simulink library "usask_tlm_lib"  (R2015a)
settings: Solver=ode45  SolverMode=SingleTasking  StartTime=0.0  StopTime=10.0  RelTol=1e-3
undefined symbols (not defined in the file): B, d, L, m_E, m_G, nu, rho
libraries: TaperedTLMElasticLib x8, transmission_lines x2
(part 1 of 2)
settings Model: Creator=tkw954  LastModifiedBy=Jeremy
settings DataIOCC: SignalLoggingSaveFormat=ModelDataLogs
settings OptimizationCC: BlockReduction=off  BooleanDataType=off
settings DebuggingCC: SaveWithParameterizedLinksMsg=none  UnderspecifiedInitializationDetection=Classic  MergeDetectMultiDrivingBlocksExec=none  SignalResolutionControl=TryResolveAllWithWarning  MultiTaskDSMMsg=warning  MultiTaskCondExecSysMsg=none  StateNameClashWarn=warning  StrictBusMsg=None
settings HardwareCC: TargetUnknown=on

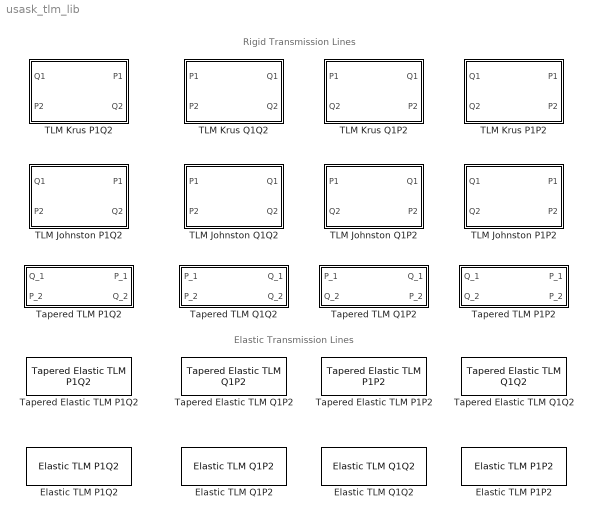
== system usask_tlm_lib ==
  note: Elastic Transmission Lines
  note: Rigid Transmission Lines
  Elastic TLM P1P2 : TaperedTLMElasticLib/Elastic TLM P1P2  K=1.5e9  nu=100e-6  rho=890  D=42e-3  L=10  e_pipe=6e-3  E=190e9  nu_p=0.3  axial_effect=Anchored throughout
  Elastic TLM P1Q2 : TaperedTLMElasticLib/Elastic TLM P1Q2  K=1.5e9  nu=100e-6  rho=890  D=42e-3  L=10  e_pipe=6e-3  E=190e9  nu_p=0.3  axial_effect=Anchored throughout
  Elastic TLM Q1P2 : TaperedTLMElasticLib/Elastic TLM Q1P2  K=1.5e9  nu=100e-6  rho=890  D=42e-3  L=10  e_pipe=6e-3  E=190e9  nu_p=0.3  axial_effect=Anchored throughout
  Elastic TLM Q1Q2 : TaperedTLMElasticLib/Elastic TLM Q1Q2  K=1.5e9  nu=100e-6  rho=890  D=42e-3  L=10  e_pipe=6e-3  E=190e9  nu_p=0.3  axial_effect=Anchored throughout
  TLM Johnston P1P2 : Subsystem  mask(Transmission Line){L=L, d=d, rho=rho, nu=nu, B=B, modelNumber=2, useCorrected=on}
      mask prompts: L "Length (m)"; d "Diameter (m)"; rho "Density (kg/m^3)"; nu "Kinematic viscosity (m^2/s)"; B "Bulk Modulus (Pa)"; modelNumber "Model Number"; useCorrected "Use corrected impedence"
      mask help:
      | Calculates pipeline dynamics using the Transmission Line Method (TLM).
      |
      | This implementation follows Johnston (2012), which includes an approximation of unsteady laminar flow and frequency-dependent velocity profile. It neglects thermal effects and assumes zero initial pressure and flow.
      |
      | Three models are implemented. Model 1 may be unstable for high beta (see paper). Model 2 is recommended.
      |
      | One may choose to use a more complicated impedence model to compensate for errors in capacitance.
      |
      | Positive flows are into both ports.
      |
      | Reference
      | Johnston, Nigel. "The transmission line method for modelling laminar flow of liquid in pipelines." Proceedings of the Institution of Mechanical Engineers, Part I: Journal of Systems and Control Engineering 226.5 (2012): 586-597.
      mask init:
      | c=sqrt(B/rho);%(m/s) sonic speed
      | 
      | A=pi/4*d^2;%(m^2) cross sectional area
      | r=d/2;%(m) radius
      | T=L/c;%(s) propagation time
      | 
      | R=8*rho*nu*L/(pi*r^4);%(Pa/(m^3/s)) Resistance
      | 
      | K=1.25;%empirical constant
      | 
      | beta=nu*T/r^2;%dissipation number
      | fprintf('beta=%f\n',beta);
      | 
      | k=4;%this must match order of G2 diagram
      | m=nan(k,1);
      | m(1)=2.2457;
      | if k>1
      | m(2)=6.8400;
      | end
      | for i=3:k
      |     m(i)=3*m(i-1);
      | end
      | 
      | 
      | n=nan(k,1);
      | n(1)=42.849;
      | for i=2:k
      |     n(i)=9*n(i-1);
      | end
      | 
      | if useCorrected
      |     Zc=rho*c/A*(1+K*(1-exp(-4*beta))+2*sum(m./n)-4*beta);%(Pa/(m^3/s)) impedence
      | else
      |     Zc=rho*c/A;%(Pa/(m^3/s)) impedence
      | end
      mask TypeOptions modelNumber: 1 | 2 | 3
  TLM Johnston P1Q2 : Subsystem  mask(Transmission Line){L=45, d=13e-3, rho=870, nu=1.2402e-04, B=1.5182e9, modelNumber=2, useCorrected=on}
      mask prompts: L "Length (m)"; d "Diameter (m)"; rho "Density (kg/m^3)"; nu "Kinematic viscosity (m^2/s)"; B "Bulk Modulus (Pa)"; modelNumber "Model Number"; useCorrected "Use corrected impedence"
      mask help:
      | Calculates pipeline dynamics using the Transmission Line Method (TLM).
      |
      | This implementation follows Johnston (2012), which includes an approximation of unsteady laminar flow and frequency-dependent velocity profile. It neglects thermal effects and assumes zero initial pressure and flow.
      |
      | Three models are implemented. Model 1 may be unstable for high beta (see paper). Model 2 is recommended.
      |
      | One may choose to use a more complicated impedence model to compensate for errors in capacitance.
      |
      | Positive flows are into both ports.
      |
      | Reference
      | Johnston, Nigel. "The transmission line method for modelling laminar flow of liquid in pipelines." Proceedings of the Institution of Mechanical Engineers, Part I: Journal of Systems and Control Engineering 226.5 (2012): 586-597.
      mask init: same as usask_tlm_lib/TLM Johnston P1P2
      mask TypeOptions modelNumber: 1 | 2 | 3
  TLM Johnston Q1P2 : Subsystem  mask(Transmission Line){L=45, d=13e-3, rho=870, nu=1.2402e-04, B=1.5182e9, modelNumber=2, useCorrected=on}
      mask prompts: L "Length (m)"; d "Diameter (m)"; rho "Density (kg/m^3)"; nu "Kinematic viscosity (m^2/s)"; B "Bulk Modulus (Pa)"; modelNumber "Model Number"; useCorrected "Use corrected impedence"
      mask help:
      | Calculates pipeline dynamics using the Transmission Line Method (TLM).
      |
      | This implementation follows Johnston (2012), which includes an approximation of unsteady laminar flow and frequency-dependent velocity profile. It neglects thermal effects and assumes zero initial pressure and flow.
      |
      | Three models are implemented. Model 1 may be unstable for high beta (see paper). Model 2 is recommended.
      |
      | One may choose to use a more complicated impedence model to compensate for errors in capacitance.
      |
      | Positive flows are into both ports.
      |
      | Reference
      | Johnston, Nigel. "The transmission line method for modelling laminar flow of liquid in pipelines." Proceedings of the Institution of Mechanical Engineers, Part I: Journal of Systems and Control Engineering 226.5 (2012): 586-597.
      mask init: same as usask_tlm_lib/TLM Johnston P1P2
      mask TypeOptions modelNumber: 1 | 2 | 3
  TLM Johnston Q1Q2 : Subsystem  mask(Transmission Line){L=45, d=13e-3, rho=870, nu=1.2402e-04, B=1.5182e9, modelNumber=2, useCorrected=on}
      mask prompts: L "Length (m)"; d "Diameter (m)"; rho "Density (kg/m^3)"; nu "Kinematic viscosity (m^2/s)"; B "Bulk Modulus (Pa)"; modelNumber "Model Number"; useCorrected "Use corrected impedence"
      mask help:
      | Calculates pipeline dynamics using the Transmission Line Method (TLM).
      |
      | This implementation follows Johnston (2012), which includes an approximation of unsteady laminar flow and frequency-dependent velocity profile. It neglects thermal effects and assumes zero initial pressure and flow.
      |
      | Three models are implemented. Model 1 may be unstable for high beta (see paper). Model 2 is recommended.
      |
      | One may choose to use a more complicated impedence model to compensate for errors in capacitance.
      |
      | Positive flows are into both ports.
      |
      | Reference
      | Johnston, Nigel. "The transmission line method for modelling laminar flow of liquid in pipelines." Proceedings of the Institution of Mechanical Engineers, Part I: Journal of Systems and Control Engineering 226.5 (2012): 586-597.
      mask init: same as usask_tlm_lib/TLM Johnston P1P2
      mask TypeOptions modelNumber: 1 | 2 | 3
  TLM Krus P1P2 : Subsystem  mask(Transmission Line){L=45, d=13e-3, rho=870, nu=1.2402e-04, B=1.5182e9}
      mask prompts: L "Length (m)"; d "Diameter (m)"; rho "Density (kg/m^3)"; nu "Kinematic viscosity (m^2/s)"; B "Bulk Modulus (Pa)"
      mask help:
      | Calculates pipeline dynamics using the Transmission Line Method (TLM).
      |
      | This implementation follows Krus et al (1994), which neglects unsteady friciton and uses simple transfer functions for the filters.
      |
      | Reference
      | Krus P, Weddfelt K and Palmberg J-O. Fast pipeline models for simulation of hydraulic systems. J Dyn Syst Measure Control 1994; 116(1): 132–136.
      mask init:
      | c=sqrt(B/rho);%(m/s) sonic speed
      | 
      | A=pi/4*d^2;%(m^2) cross sectional area
      | r=d/2;%(m) radius
      | T=L/c;%(s) propagation time
      | 
      | R=8*rho*nu*L/(pi*r^4);%(Pa/(m^3/s)) Resistance
      | 
      | K=1.25;%empirical constant
      | 
      | Zc=rho*c/A;%(Pa/(m^3/s)) impedence
      | 
      | beta=nu*T/r^2;%dissipation number
      | fprintf('beta=%f\n',beta);
  TLM Krus P1Q2 : Subsystem  mask(Transmission Line){L=45, d=13e-3, rho=870, nu=1.2402e-04, B=1.5182e9}
      mask prompts: L "Length (m)"; d "Diameter (m)"; rho "Density (kg/m^3)"; nu "Kinematic viscosity (m^2/s)"; B "Bulk Modulus (Pa)"
      mask help:
      | Calculates pipeline dynamics using the Transmission Line Method (TLM).
      |
      | This implementation follows Krus et al (1994), which neglects unsteady friciton and uses simple transfer functions for the filters.
      |
      | Reference
      | Krus P, Weddfelt K and Palmberg J-O. Fast pipeline models for simulation of hydraulic systems. J Dyn Syst Measure Control 1994; 116(1): 132–136.
      mask init: same as usask_tlm_lib/TLM Krus P1P2
  TLM Krus Q1P2 : Subsystem  mask(Transmission Line){L=45, d=13e-3, rho=870, nu=1.2402e-04, B=1.5182e9}
      mask prompts: L "Length (m)"; d "Diameter (m)"; rho "Density (kg/m^3)"; nu "Kinematic viscosity (m^2/s)"; B "Bulk Modulus (Pa)"
      mask help:
      | Calculates pipeline dynamics using the Transmission Line Method (TLM).
      |
      | This implementation follows Krus et al (1994), which neglects unsteady friciton and uses simple transfer functions for the filters.
      |
      | Reference
      | Krus P, Weddfelt K and Palmberg J-O. Fast pipeline models for simulation of hydraulic systems. J Dyn Syst Measure Control 1994; 116(1): 132–136.
      mask init: same as usask_tlm_lib/TLM Krus P1P2
  TLM Krus Q1Q2 : Subsystem  mask(Transmission Line){L=45, d=13e-3, rho=870, nu=1.2402e-04, B=1.5182e9}
      mask prompts: L "Length (m)"; d "Diameter (m)"; rho "Density (kg/m^3)"; nu "Kinematic viscosity (m^2/s)"; B "Bulk Modulus (Pa)"
      mask help:
      | Calculates pipeline dynamics using the Transmission Line Method (TLM).
      |
      | This implementation follows Krus et al (1994), which neglects unsteady friciton and uses simple transfer functions for the filters.
      |
      | Reference
      | Krus P, Weddfelt K and Palmberg J-O. Fast pipeline models for simulation of hydraulic systems. J Dyn Syst Measure Control 1994; 116(1): 132–136.
      mask init: same as usask_tlm_lib/TLM Krus P1P2
  Tapered Elastic TLM P1P2 : TaperedTLMElasticLib/Tapered Elastic TLM P1P2  K=1.5e9  nu=100e-6  rho=890  D_1=40e-3  D_2=42e-3  L=10  e_pipe=3e-3  E=2e9  nu_p=0.3  axial_effect=Anchored throughout
  Tapered Elastic TLM P1Q2 : TaperedTLMElasticLib/Tapered Elastic TLM P1Q2  K=1.5e9  nu=100e-6  rho=890  D_1=40e-3  D_2=42e-3  L=10  e_pipe=3e-3  E=2e9  nu_p=0.3  axial_effect=Anchored throughout
  Tapered Elastic TLM Q1P2 : TaperedTLMElasticLib/Tapered Elastic TLM Q1P2  K=1.5e9  nu=100e-6  rho=890  D_1=40e-3  D_2=42e-3  L=10  e_pipe=3e-3  E=2e9  nu_p=0.3  axial_effect=Anchored throughout
  Tapered Elastic TLM Q1Q2 : TaperedTLMElasticLib/Tapered Elastic TLM Q1Q2  K=1.5e9  nu=100e-6  rho=890  D_1=40e-3  D_2=42e-3  L=10  e_pipe=3e-3  E=2e9  nu_p=0.3  axial_effect=Anchored throughout
  Tapered TLM P1P2 : Subsystem  mask(Tapered Hydraulic Transmission Line (TLM)){D_1=40e-3, D_2=42e-3, L=10, K=1.5e9, nu=100e-6, rho=890}
      mask prompts: D_1 "Inlet Diameter (m)"; D_2 "Outlet Diameter (m)"; L "Length (m)"; K "Oil Bulk Modulus (Pa)"; nu "Oil Viscosity (m^2/s)"; rho "Oil Density (kg/m^3)"
      mask help:
      | This model implements the transmission line model in ven der Buhs and Wiens (2017). The method uses the the transfer function form from Johnston et. al (2014), however the weighting factors are determined from an optimization procedure comparing to the exact transmission matrix for a tapered pipeline.
      |
      | This model assumes a rigid-walled tube with a linear taper in radius between the two ports. It assumes constant bulk modulus (no cavitation or entrined air effects) and includes frequency-dependent friction effects.
      |
      | Positive flows are directed into either port.
      |
      | This model also assumes zero initial conditions
      |
      | Reference:
      | N Johnston, M Pan, and S Kudzma. An enhanced transmission line method for modelling laminar flow of liquid in pipelines. Journal of Systems and Control Engineering, 228(4):193–206, 2014.
      |
      | J ven der Buhs and T Wiens. Modelling Dynamic Response of Hydraulic Fluid Within Tapered Transmission Lines. Proceedings of the 15th Scandinavian International Conference on Fluid Power, 2017
      mask init:
      | %% Note: Equation numbers from:
      | % J ven der Buhs and T Wiens. Modelling Dynamic Response of Hydraulic Fluid Within Tapered 
      | % Transmission Lines. Proceedings of the 15th Scandinavian International Conference on Fluid 
      | % Power, Linköping University, Sweden, 2017.
      | %%
      | 
      | % Check for positive params, report error if negative given
      | if D_1<0 | D_2<0 | L<0 | K<0 | nu<0 | rho<0
      |     error('Please ensure parameters are all positive')
      | end
      | 
      | r1 = D_1/2; % Inlet radius (m)
      | r2 = D_2/2; % Outlet radius (m)
      | 
      | c=sqrt(K/rho);% Local speed of sound (m/s)
      | lambda = min(r1,r2)/max(r1,r2); % Taper ratio (dimensionless), Equation (11)
      | beta = ((nu*L)/(c*max(r1,r2)^2))*((lambda^2+lambda+1)^2/(9*lambda^3)); % Dissipation number (dimensionless), Equation (13)
      | Z_c = ((3*c*rho)/(pi*max(r1,r2)^2))/(lambda^2+lambda+1); % Characteristic impedance (Pa•s/m^3), Equation (10)
      | T=L/c; % Wave propagation time (s)
      | 
      | k=6; % Number of weighting factors
      | 
      | % Grab optimized weighting factors and parameters. Please see paper for
      | % more detail on how these parameters were found.
      | [ m_E, m_G, tau ] = interpolateTLMparams( beta, lambda, k);
      | 
      | if isnan(m_E(1)) | isnan(m_G(1)) | isnan(tau)
      |     error('The parameters you have entered are outside the working range of this model. Weighting factors cannot be found')
      | end  
      |     
      | T_prime = tau*T; % Modified wave propagation time (s), Equation (18) 
      | 
      | n=nan(1,k); % Weighting factor initialization
      | n(1)=0.3/(1+3*beta); % Equation (19)
      | for i=2:k
      |     n(i)=n(i-1)*3; % Equation (19)
      | end
      | 
      | b=1-8*beta/sum(m_E./n); % Equation (16)
      | 
      | %Error Checking
      | load TaperedTLMAcceptableErrorContour.mat
      | IN = inpolygon(lambda,beta,lambda_poly,beta_poly);
      | if ~IN
      |     warning('Dissipaton number (beta) and taper ratio (lambda) combination are outside the recommended range')
      | end
      | 
      | 
      | 
      | 
      | %% End of initialization
      mask Display:
      | port_label('input', 1 , '\itq_1', 'texmode', 'on')
      | port_label('input', 2 , '\itq_2', 'texmode', 'on')
      | port_label('output', 1 , '\itp_1', 'texmode', 'on')
      | port_label('output', 2 , '\itp_2', 'texmode', 'on')
  Tapered TLM P1Q2 : Subsystem  mask(Tapered Hydraulic Transmission Line (TLM)){D_1=40e-3, D_2=42e-3, L=10, K=1.5e9, nu=100e-6, rho=890}
      mask prompts: D_1 "Inlet Diameter (m)"; D_2 "Outlet Diameter (m)"; L "Length (m)"; K "Oil Bulk Modulus (Pa)"; nu "Oil Viscosity (m^2/s)"; rho "Oil Density (kg/m^3)"
      mask help:
      | This model implements the transmission line model in ven der Buhs and Wiens (2017). The method uses the the transfer function form from Johnston et. al (2014), however the weighting factors are determined from an optimization procedure comparing to the exact transmission matrix for a tapered pipeline.
      |
      | This model assumes a rigid-walled tube with a linear taper in radius between the two ports. It assumes constant bulk modulus (no cavitation or entrined air effects) and includes frequency-dependent friction effects.
      |
      | Positive flows are directed into either port. This model also assumes zero initial conditions.
      |
      | "p" is fluid pressure in pascals (Pa).
      | "q" is fluid flow in cubic meters per second (m^3/s).
      | "_1" indicates the inlet, and "_2" indicates the outlet.
      |
      | Reference:
      | N Johnston, M Pan, and S Kudzma. An enhanced transmission line method for modelling laminar flow of liquid in pipelines. Journal of Systems and Control Engineering, 228(4):193–206, 2014.
      |
      | J ven der Buhs and T Wiens. Modelling Dynamic Response of Hydraulic Fluid Within Tapered Transmission Lines. Proceedings of the 15th Scandinavian International Conference on Fluid Power, Linköping University, Sweden, 2017.
      mask init: same as usask_tlm_lib/Tapered TLM P1P2
      mask Display:
      | port_label('input', 1 , '\itq_1', 'texmode', 'on')
      | port_label('input', 2 , '\itp_2', 'texmode', 'on')
      | port_label('output', 1 , '\itp_1', 'texmode', 'on')
      | port_label('output', 2 , '\itq_2', 'texmode', 'on')
  Tapered TLM Q1P2 : Subsystem  mask(Tapered Hydraulic Transmission Line (TLM)){D_1=40e-3, D_2=42e-3, L=10, K=1.5e9, nu=100e-6, rho=890}
      mask prompts: D_1 "Inlet Diameter (m)"; D_2 "Outlet Diameter (m)"; L "Length (m)"; K "Oil Bulk Modulus (Pa)"; nu "Oil Viscosity (m^2/s)"; rho "Oil Density (kg/m^3)"
      mask help:
      | This model implements the transmission line model in ven der Buhs and Wiens (2017). The method uses the the transfer function form from Johnston et. al (2014), however the weighting factors are determined from an optimization procedure comparing to the exact transmission matrix for a tapered pipeline.
      |
      | This model assumes a rigid-walled tube with a linear taper in radius between the two ports. It assumes constant bulk modulus (no cavitation or entrined air effects) and includes frequency-dependent friction effects.
      |
      | Positive flows are directed into either port.
      |
      | This model also assumes zero initial conditions
      |
      | Reference:
      | N Johnston, M Pan, and S Kudzma. An enhanced transmission line method for modelling laminar flow of liquid in pipelines. Journal of Systems and Control Engineering, 228(4):193–206, 2014.
      |
      | J ven der Buhs and T Wiens. Modelling Dynamic Response of Hydraulic Fluid Within Tapered Transmission Lines. Proceedings of the 15th Scandinavian International Conference on Fluid Power, 2017
      mask init: same as usask_tlm_lib/Tapered TLM P1P2
      mask Display:
      | port_label('input', 1 , '\itp_1', 'texmode', 'on')
      | port_label('input', 2 , '\itq_2', 'texmode', 'on')
      | port_label('output', 1 , '\itq_1', 'texmode', 'on')
      | port_label('output', 2 , '\itp_2', 'texmode', 'on')
  Tapered TLM Q1Q2 : Subsystem  mask(Tapered Hydraulic Transmission Line (TLM)){D_1=40e-3, D_2=42e-3, L=10, K=1.5e9, nu=100e-6, rho=890}
      mask prompts: D_1 "Inlet Diameter (m)"; D_2 "Outlet Diameter (m)"; L "Length (m)"; K "Oil Bulk Modulus (Pa)"; nu "Oil Viscosity (m^2/s)"; rho "Oil Density (kg/m^3)"
      mask help:
      | This model implements the transmission line model in ven der Buhs and Wiens (2017). The method uses the the transfer function form from Johnston et. al (2014), however the weighting factors are determined from an optimization procedure comparing to the exact transmission matrix for a tapered pipeline.
      |
      | This model assumes a rigid-walled tube with a linear taper in radius between the two ports. It assumes constant bulk modulus (no cavitation or entrined air effects) and includes frequency-dependent friction effects.
      |
      | Positive flows are directed into either port.
      |
      | This model also assumes zero initial conditions
      |
      | Reference:
      | N Johnston, M Pan, and S Kudzma. An enhanced transmission line method for modelling laminar flow of liquid in pipelines. Journal of Systems and Control Engineering, 228(4):193–206, 2014.
      |
      | J ven der Buhs and T Wiens. Modelling Dynamic Response of Hydraulic Fluid Within Tapered Transmission Lines. Proceedings of the 15th Scandinavian International Conference on Fluid Power, 2017
      mask init: same as usask_tlm_lib/Tapered TLM P1P2
      mask Display:
      | port_label('input', 1 , '\itp_1', 'texmode', 'on')
      | port_label('input', 2 , '\itp_2', 'texmode', 'on')
      | port_label('output', 1 , '\itq_1', 'texmode', 'on')
      | port_label('output', 2 , '\itq_2', 'texmode', 'on')

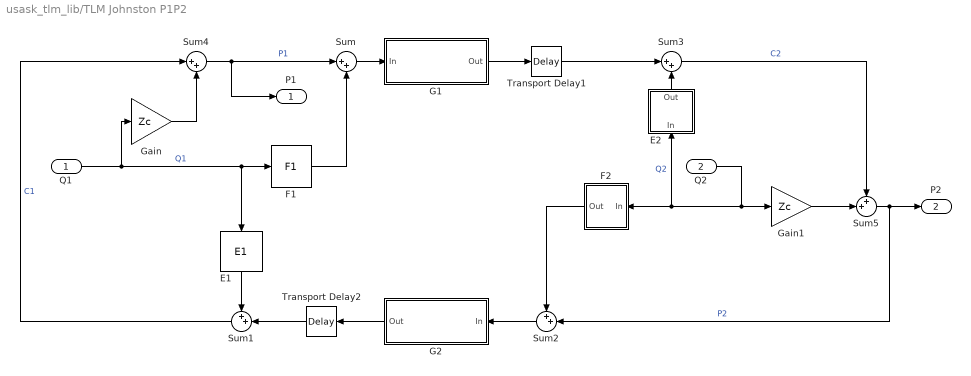
== system usask_tlm_lib/TLM Johnston P1P2 ==
  Q1 : Inport
  Q2 : Inport  Port=2
  E1 : transmission_lines/TLM Krus P1P2/E1
  E2 : Subsystem
  F1 : transmission_lines/TLM Krus P1P2/F1
  F2 : Subsystem
  G1 : Subsystem
  G2 : Subsystem
  Gain : Gain  Gain=Zc
  Gain1 : Gain  Gain=Zc
  Sum : Sum  Inputs=|++
  Sum1 : Sum  Inputs=++|
  Sum2 : Sum  Inputs=++|
  Sum3 : Sum  Inputs=|++
  Sum4 : Sum  Inputs=|++
  Sum5 : Sum  Inputs=++|
  Transport Delay1 : TransportDelay  DelayTime=T
  Transport Delay2 : TransportDelay  DelayTime=T
  P1 : Outport
  P2 : Outport  Port=2
  wires:
  Sum3/1 -> Sum5/1  "C2"
  G1/1(Out) -> Transport Delay1/1
  E2/1(Out) -> Sum3/2
  Sum5/1 -> Sum2/2, P2/1  "P2"
  Sum2/1 -> G2/1(In)
  F2/1(Out) -> Sum2/1
  Q2/1 -> F2/1(In), E2/1(In), Gain1/1  "Q2"
  Transport Delay1/1 -> Sum3/1
  Gain1/1 -> Sum5/2
  Sum/1 -> G1/1(In)
  Transport Delay2/1 -> Sum1/2
  Sum1/1 -> Sum4/1  "C1"
  F1/1 -> Sum/2
  E1/1 -> Sum1/1
  G2/1(Out) -> Transport Delay2/1
  Q1/1 -> Gain/1, F1/1, E1/1  "Q1"
  Sum4/1 -> P1/1, Sum/1  "P1"
  Gain/1 -> Sum4/2

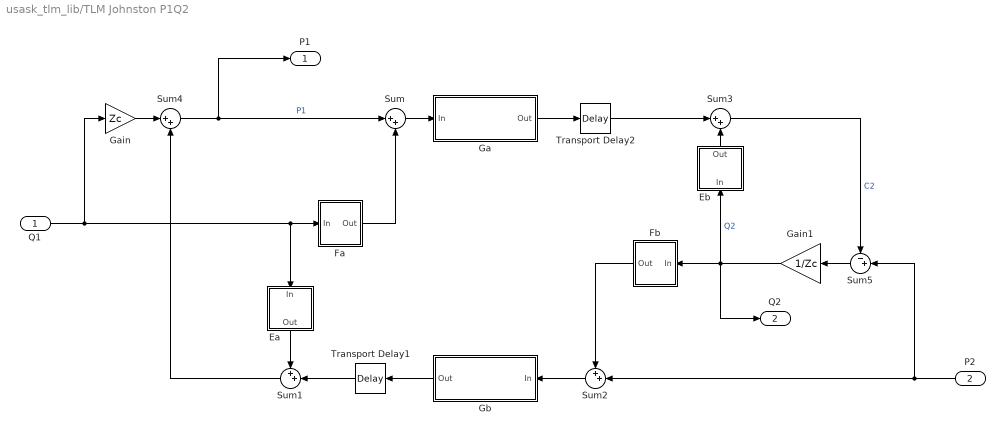
== system usask_tlm_lib/TLM Johnston P1Q2 ==
  Q1 : Inport
  P2 : Inport  Port=2
  Ea : Subsystem
  Eb : Subsystem
  Fa : Subsystem
  Fb : Subsystem
  Ga : Subsystem
  Gain : Gain  Gain=Zc
  Gain1 : Gain  Gain=1/Zc
  Gb : Subsystem
  Sum : Sum  Inputs=|++
  Sum1 : Sum  Inputs=++|
  Sum2 : Sum  Inputs=++|
  Sum3 : Sum  Inputs=|++
  Sum4 : Sum  Inputs=|++
  Sum5 : Sum  Inputs=-+|
  Transport Delay1 : TransportDelay  DelayTime=T
  Transport Delay2 : TransportDelay  DelayTime=T
  P1 : Outport
  Q2 : Outport  Port=2
  wires:
  Sum4/1 -> P1/1, Sum/1  "P1"
  Sum/1 -> Ga/1(In)
  Transport Delay2/1 -> Sum3/1
  Gain/1 -> Sum4/1
  Sum5/1 -> Gain1/1
  Transport Delay1/1 -> Sum1/2
  Q1/1 -> Gain/1, Ea/1(In), Fa/1(In)
  Sum1/1 -> Sum4/2
  Fa/1(Out) -> Sum/2
  Gain1/1 -> Q2/1, Eb/1(In), Fb/1(In)  "Q2"
  Fb/1(Out) -> Sum2/1
  Sum2/1 -> Gb/1(In)
  Ea/1(Out) -> Sum1/1
  Gb/1(Out) -> Transport Delay1/1
  P2/1 -> Sum5/2, Sum2/2
  Eb/1(Out) -> Sum3/2
  Ga/1(Out) -> Transport Delay2/1
  Sum3/1 -> Sum5/1  "C2"

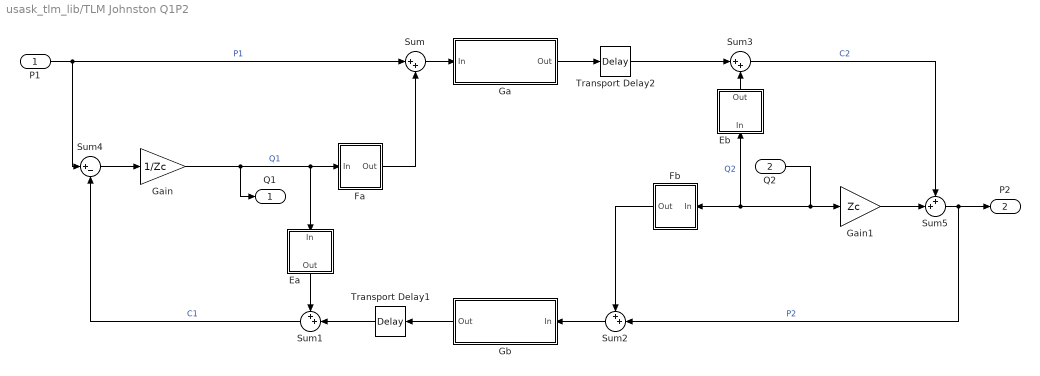
== system usask_tlm_lib/TLM Johnston Q1P2 ==
  P1 : Inport
  Q2 : Inport  Port=2
  Ea : Subsystem
  Eb : Subsystem
  Fa : Subsystem
  Fb : Subsystem
  Ga : Subsystem
  Gain : Gain  Gain=1/Zc
  Gain1 : Gain  Gain=Zc
  Gb : Subsystem
  Sum : Sum  Inputs=|++
  Sum1 : Sum  Inputs=++|
  Sum2 : Sum  Inputs=++|
  Sum3 : Sum  Inputs=|++
  Sum4 : Sum  Inputs=|+-
  Sum5 : Sum  Inputs=++|
  Transport Delay1 : TransportDelay  DelayTime=T
  Transport Delay2 : TransportDelay  DelayTime=T
  Q1 : Outport
  P2 : Outport  Port=2
  wires:
  Gain1/1 -> Sum5/2
  P1/1 -> Sum4/1, Sum/1  "P1"
  Sum/1 -> Ga/1(In)
  Transport Delay2/1 -> Sum3/1
  Transport Delay1/1 -> Sum1/2
  Gain/1 -> Q1/1, Ea/1(In), Fa/1(In)  "Q1"
  Sum1/1 -> Sum4/2  "C1"
  Fa/1(Out) -> Sum/2
  Q2/1 -> Gain1/1, Eb/1(In), Fb/1(In)  "Q2"
  Fb/1(Out) -> Sum2/1
  Sum2/1 -> Gb/1(In)
  Ea/1(Out) -> Sum1/1
  Gb/1(Out) -> Transport Delay1/1
  Sum5/1 -> P2/1, Sum2/2  "P2"
  Eb/1(Out) -> Sum3/2
  Ga/1(Out) -> Transport Delay2/1
  Sum3/1 -> Sum5/1  "C2"
  Sum4/1 -> Gain/1

== system usask_tlm_lib/TLM Johnston Q1Q2 ==
  P1 : Inport
  P2 : Inport  Port=2
  Ea : Subsystem
  Eb : Subsystem
  Fa : Subsystem
  Fb : Subsystem
  Ga : Subsystem
  Gain : Gain  Gain=1/Zc
  Gain1 : Gain  Gain=1/Zc
  Gb : Subsystem
  Sum : Sum  Inputs=|++
  Sum1 : Sum  Inputs=++|
  Sum2 : Sum  Inputs=++|
  Sum3 : Sum  Inputs=|++
  Sum4 : Sum  Inputs=|+-
  Sum5 : Sum  Inputs=-+|
  Transport Delay1 : TransportDelay  DelayTime=T
  Transport Delay2 : TransportDelay  DelayTime=T
  Q1 : Outport
  Q2 : Outport  Port=2
  wires:
  P1/1 -> Sum4/1, Sum/1  "P1"
  Sum/1 -> Ga/1(In)
  Transport Delay2/1 -> Sum3/1
  Sum5/1 -> Gain1/1
  Transport Delay1/1 -> Sum1/2
  Gain/1 -> Q1/1, Ea/1(In), Fa/1(In)  "Q1"
  Sum1/1 -> Sum4/2  "C1"
  Fa/1(Out) -> Sum/2
  Gain1/1 -> Q2/1, Eb/1(In), Fb/1(In)  "Q2"
  Fb/1(Out) -> Sum2/1
  Sum2/1 -> Gb/1(In)
  Ea/1(Out) -> Sum1/1
  Gb/1(Out) -> Transport Delay1/1
  P2/1 -> Sum5/2, Sum2/2
  Eb/1(Out) -> Sum3/2
  Ga/1(Out) -> Transport Delay2/1
  Sum3/1 -> Sum5/1  "C2"
  Sum4/1 -> Gain/1

== system usask_tlm_lib/TLM Krus P1P2 ==
  Q1 : Inport
  Q2 : Inport  Port=2
  E1 : Subsystem
  E2 : Subsystem
  F1 : Subsystem
  F2 : Subsystem
  G1 : Subsystem
  G2 : Subsystem
  Gain : Gain  Gain=Zc
  Gain1 : Gain  Gain=Zc
  Sum : Sum  Inputs=|++
  Sum1 : Sum  Inputs=++|
  Sum2 : Sum  Inputs=++|
  Sum3 : Sum  Inputs=|++
  Sum4 : Sum  Inputs=|++
  Sum5 : Sum  Inputs=++|
  Transport Delay1 : TransportDelay  DelayTime=T
  Transport Delay2 : TransportDelay  DelayTime=T
  P1 : Outport
  P2 : Outport  Port=2
  wires:
  Gain/1 -> Sum4/2
  Sum4/1 -> Sum/1, P1/1  "P1"
  Q1/1 -> E1/1(In), F1/1(In), Gain/1  "Q1"
  Sum3/1 -> Sum5/1  "C2"
  Sum5/1 -> P2/1, Sum2/2  "P2"
  Q2/1 -> E2/1(In), F2/1(In), Gain1/1  "Q2"
  Gain1/1 -> Sum5/2
  G1/1(Out) -> Transport Delay2/1
  E2/1(Out) -> Sum3/2
  G2/1(Out) -> Transport Delay1/1
  E1/1(Out) -> Sum1/1
  Sum2/1 -> G2/1(In)
  F2/1(Out) -> Sum2/1
  F1/1(Out) -> Sum/2
  Sum1/1 -> Sum4/1  "C1"
  Transport Delay1/1 -> Sum1/2
  Transport Delay2/1 -> Sum3/1
  Sum/1 -> G1/1(In)

== system usask_tlm_lib/TLM Krus P1Q2 ==
  Q1 : Inport
  P2 : Inport  Port=2
  E1 : Subsystem
  E2 : Subsystem
  F1 : Subsystem
  F2 : Subsystem
  G1 : Subsystem
  G2 : Subsystem
  Gain : Gain  Gain=Zc
  Gain1 : Gain  Gain=1/Zc
  Sum : Sum  Inputs=|++
  Sum1 : Sum  Inputs=++|
  Sum2 : Sum  Inputs=++|
  Sum3 : Sum  Inputs=|++
  Sum4 : Sum  Inputs=|++
  Sum5 : Sum  Inputs=-+|
  Transport Delay1 : TransportDelay  DelayTime=T
  Transport Delay2 : TransportDelay  DelayTime=T
  P1 : Outport
  Q2 : Outport  Port=2
  wires:
  Sum4/1 -> P1/1, Sum/1  "P1"
  Sum/1 -> G1/1(In)
  Transport Delay2/1 -> Sum3/1
  Gain/1 -> Sum4/1
  Sum5/1 -> Gain1/1
  Transport Delay1/1 -> Sum1/2
  Q1/1 -> Gain/1, E1/1(In), F1/1(In)
  Sum1/1 -> Sum4/2
  F1/1(Out) -> Sum/2
  Gain1/1 -> Q2/1, E2/1(In), F2/1(In)  "Q2"
  F2/1(Out) -> Sum2/1
  Sum2/1 -> G2/1(In)
  E1/1(Out) -> Sum1/1
  G2/1(Out) -> Transport Delay1/1
  P2/1 -> Sum5/2, Sum2/2
  E2/1(Out) -> Sum3/2
  G1/1(Out) -> Transport Delay2/1
  Sum3/1 -> Sum5/1  "C2"

== system usask_tlm_lib/TLM Krus Q1P2 ==
  P1 : Inport
  Q2 : Inport  Port=2
  E1 : Subsystem
  E2 : Subsystem
  F1 : Subsystem
  F2 : Subsystem
  G1 : Subsystem
  G2 : Subsystem
  Gain : Gain  Gain=1/Zc
  Gain1 : Gain  Gain=Zc
  Sum : Sum  Inputs=|++
  Sum1 : Sum  Inputs=++|
  Sum2 : Sum  Inputs=++|
  Sum3 : Sum  Inputs=|++
  Sum4 : Sum  Inputs=|+-
  Sum5 : Sum  Inputs=++|
  Transport Delay1 : TransportDelay  DelayTime=T
  Transport Delay2 : TransportDelay  DelayTime=T
  Q1 : Outport
  P2 : Outport  Port=2
  wires:
  Sum3/1 -> Sum5/1  "C2"
  Sum5/1 -> P2/1, Sum2/2  "P2"
  Q2/1 -> E2/1(In), F2/1(In), Gain1/1  "Q2"
  Gain1/1 -> Sum5/2
  Sum4/1 -> Gain/1
  G1/1(Out) -> Transport Delay2/1
  E2/1(Out) -> Sum3/2
  G2/1(Out) -> Transport Delay1/1
  E1/1(Out) -> Sum1/1
  Sum2/1 -> G2/1(In)
  F2/1(Out) -> Sum2/1
  F1/1(Out) -> Sum/2
  Sum1/1 -> Sum4/2  "C1"
  Gain/1 -> Q1/1, E1/1(In), F1/1(In)  "Q1"
  Transport Delay1/1 -> Sum1/2
  Transport Delay2/1 -> Sum3/1
  Sum/1 -> G1/1(In)
  P1/1 -> Sum4/1, Sum/1  "P1"

== system usask_tlm_lib/TLM Krus Q1Q2 ==
  P1 : Inport
  P2 : Inport  Port=2
  E1 : Subsystem
  E2 : Subsystem
  F1 : Subsystem
  F2 : Subsystem
  G1 : Subsystem
  G2 : Subsystem
  Gain : Gain  Gain=1/Zc
  Gain1 : Gain  Gain=1/Zc
  Sum : Sum  Inputs=|++
  Sum1 : Sum  Inputs=++|
  Sum2 : Sum  Inputs=++|
  Sum3 : Sum  Inputs=|++
  Sum4 : Sum  Inputs=|+-
  Sum5 : Sum  Inputs=-+|
  Transport Delay1 : TransportDelay  DelayTime=T
  Transport Delay2 : TransportDelay  DelayTime=T
  Q1 : Outport
  Q2 : Outport  Port=2
  wires:
  Sum4/1 -> Gain/1
  Sum3/1 -> Sum5/1  "C2"
  G1/1(Out) -> Transport Delay2/1
  E2/1(Out) -> Sum3/2
  P2/1 -> Sum2/2, Sum5/2
  G2/1(Out) -> Transport Delay1/1
  E1/1(Out) -> Sum1/1
  Sum2/1 -> G2/1(In)
  F2/1(Out) -> Sum2/1
  Gain1/1 -> F2/1(In), E2/1(In), Q2/1  "Q2"
  F1/1(Out) -> Sum/2
  Sum1/1 -> Sum4/2  "C1"
  Gain/1 -> Q1/1, E1/1(In), F1/1(In)  "Q1"
  Transport Delay1/1 -> Sum1/2
  Sum5/1 -> Gain1/1
  Transport Delay2/1 -> Sum3/1
  Sum/1 -> G1/1(In)
  P1/1 -> Sum4/1, Sum/1  "P1"

== system usask_tlm_lib/Tapered TLM P1P2 ==
  Q_1 : Inport
  Q_2 : Inport  Port=2
  "  Delay_2 " : Subsystem
      mask Display: disp('\fontname{Times New Roman}\ite^{-j\omegaT}', 'texmode', 'on')
  "Delay_1 " : Subsystem
      mask Display: disp('\fontname{Times New Roman}\ite^{-j\omegaT}', 'texmode', 'on')
  E_1 : Subsystem
      mask Display: disp('\fontname{Times New Roman}\fontsize{30}\itE', 'texmode', 'on')
  E_2 : Subsystem
      mask Display: disp('\fontname{Times New Roman}\fontsize{30}\itE', 'texmode', 'on')
  F_1 : Subsystem
      mask Display: disp('\fontname{Times New Roman}\fontsize{30}\itF', 'texmode', 'on')
  F_2 : Subsystem
      mask Display: disp('\fontname{Times New Roman}\fontsize{30}\itF', 'texmode', 'on')
  G_1 : Subsystem
      mask Display: disp('\fontname{Times New Roman}\fontsize{30}\itG', 'texmode', 'on')
  G_2 : Subsystem
      mask Display: disp('\fontname{Times New Roman}\fontsize{30}\itG', 'texmode', 'on')
  Gain1 : Gain  Gain=Z_c
  Gain2 : Gain  Gain=Z_c
  Sum : Sum  Inputs=|++
  Sum1 : Sum  Inputs=|++
  Sum2 : Sum  Inputs=++|
  Sum3 : Sum  Inputs=++|
  Sum4 : Sum  Inputs=|++
  Sum5 : Sum  Inputs=++|
  P_1 : Outport
  P_2 : Outport  Port=2
  wires:
  Sum5/1 -> Sum3/2, P_2/1
  Gain2/1 -> Sum5/2
  Sum1/1 -> Sum5/1
  F_1/1(Out1) -> Sum/2
  Gain1/1 -> Sum4/1
  Q_2/1 -> E_2/1(Q_2), F_2/2(Q_2), Gain2/1
  "  Delay_2 "/1(delay) -> Sum2/2
  "Delay_1 "/1(delay) -> Sum1/1
  Sum2/1 -> Sum4/2
  F_2/1(F) -> Sum3/1
  Sum3/1 -> G_2/1(F + P_2)
  Sum4/1 -> Sum/1, P_1/1
  Q_1/1 -> E_1/1(Q_1), F_1/1(Q_1), Gain1/1
  G_2/1(G) -> "  Delay_2 "/1(G)
  E_1/1(E) -> Sum2/1, F_1/2(E)
  E_2/1(E) -> F_2/1(E), Sum1/2
  G_1/1(G) -> "Delay_1 "/1(G)
  Sum/1 -> G_1/1(F + P_1)

== system usask_tlm_lib/Tapered TLM P1Q2 ==
  Q_1 : Inport
  P_2 : Inport  Port=2
  "  Delay_2 " : Subsystem
      mask Display: disp('\fontname{Times New Roman}\ite^{-j\omegaT}', 'texmode', 'on')
  "Delay_1 " : Subsystem
      mask Display: disp('\fontname{Times New Roman}\ite^{-j\omegaT}', 'texmode', 'on')
  E_1 : Subsystem
      mask Display: disp('\fontname{Times New Roman}\fontsize{30}\itE', 'texmode', 'on')
  E_2 : Subsystem
      mask Display: disp('\fontname{Times New Roman}\fontsize{30}\itE', 'texmode', 'on')
  F_1 : Subsystem
      mask Display: disp('\fontname{Times New Roman}\fontsize{30}\itF', 'texmode', 'on')
  F_2 : Subsystem
      mask Display: disp('\fontname{Times New Roman}\fontsize{30}\itF', 'texmode', 'on')
  G_1 : Subsystem
      mask Display: disp('\fontname{Times New Roman}\fontsize{30}\itG', 'texmode', 'on')
  G_2 : Subsystem
      mask Display: disp('\fontname{Times New Roman}\fontsize{30}\itG', 'texmode', 'on')
  Gain1 : Gain  Gain=Z_c
  Gain3 : Gain  Gain=1/Z_c
  Sum : Sum  Inputs=|++
  Sum1 : Sum  Inputs=|++
  Sum2 : Sum  Inputs=++|
  Sum3 : Sum  Inputs=++|
  Sum4 : Sum  Inputs=|++
  Sum5 : Sum  Inputs=-+|
  P_1 : Outport
  Q_2 : Outport  Port=2
  wires:
  F_1/1(F) -> Sum/2
  Sum5/1 -> Gain3/1
  Gain1/1 -> Sum4/1
  Gain3/1 -> Q_2/1, E_2/1(Q_2), F_2/2(Q_2)
  "  Delay_2 "/1(delay) -> Sum2/2
  "Delay_1 "/1(delay) -> Sum1/1
  P_2/1 -> Sum3/2, Sum5/2
  Sum1/1 -> Sum5/1
  Sum2/1 -> Sum4/2
  F_2/1(Out1) -> Sum3/1
  Sum3/1 -> G_2/1(F + P_2)
  Sum4/1 -> Sum/1, P_1/1
  Q_1/1 -> E_1/1(Q_1), F_1/1(Q_1), Gain1/1
  G_2/1(G) -> "  Delay_2 "/1(G)
  E_1/1(E) -> Sum2/1, F_1/2(E)
  E_2/1(E) -> F_2/1(E), Sum1/2
  G_1/1(G) -> "Delay_1 "/1(G)
  Sum/1 -> G_1/1(F + P_1)

== system usask_tlm_lib/Tapered TLM Q1P2 ==
  P_1 : Inport
  Q_2 : Inport  Port=2
  "  Delay_2 " : Subsystem
      mask Display: disp('\fontname{Times New Roman}\ite^{-j\omegaT}', 'texmode', 'on')
  "Delay_1 " : Subsystem
      mask Display: disp('\fontname{Times New Roman}\ite^{-j\omegaT}', 'texmode', 'on')
  E_1 : Subsystem
      mask Display: disp('\fontname{Times New Roman}\fontsize{30}\itE', 'texmode', 'on')
  E_2 : Subsystem
      mask Display: disp('\fontname{Times New Roman}\fontsize{30}\itE', 'texmode', 'on')
  F_1 : Subsystem
      mask Display: disp('\fontname{Times New Roman}\fontsize{30}\itF', 'texmode', 'on')
  F_2 : Subsystem
      mask Display: disp('\fontname{Times New Roman}\fontsize{30}\itF', 'texmode', 'on')
  G_1 : Subsystem
      mask Display: disp('\fontname{Times New Roman}\fontsize{30}\itG', 'texmode', 'on')
  G_2 : Subsystem
      mask Display: disp('\fontname{Times New Roman}\fontsize{30}\itG', 'texmode', 'on')
  Gain1 : Gain  Gain=Z_c
  Gain2 : Gain  Gain=1/Z_c
  Sum : Sum  Inputs=|++
  Sum1 : Sum  Inputs=|++
  Sum2 : Sum  Inputs=++|
  Sum3 : Sum  Inputs=++|
  Sum4 : Sum  Inputs=++|
  Sum6 : Sum  Inputs=|+-
  Q_1 : Outport
  P_2 : Outport  Port=2
  wires:
  Gain1/1 -> Sum4/2
  Sum4/1 -> Sum3/2, P_2/1
  Sum1/1 -> Sum4/1
  Sum2/1 -> Sum6/2
  Gain2/1 -> E_1/1(Q_1), F_1/1(Q_1), Q_1/1
  Sum6/1 -> Gain2/1
  F_1/1(F) -> Sum/2
  Q_2/1 -> E_2/1(Q_2), F_2/2(Q_2), Gain1/1
  "  Delay_2 "/1(delay) -> Sum2/2
  "Delay_1 "/1(delay) -> Sum1/1
  F_2/1(Out1) -> Sum3/1
  Sum3/1 -> G_2/1(F + P_2)
  P_1/1 -> Sum/1, Sum6/1
  G_2/1(G) -> "  Delay_2 "/1(G)
  E_1/1(E) -> Sum2/1, F_1/2(E)
  E_2/1(E) -> F_2/1(E), Sum1/2
  G_1/1(G) -> "Delay_1 "/1(G)
  Sum/1 -> G_1/1(F + P_1)

== system usask_tlm_lib/Tapered TLM Q1Q2 ==
  P_1 : Inport
  P_2 : Inport  Port=2
  "  Delay_2 " : Subsystem
      mask Display: disp('\fontname{Times New Roman}\ite^{-j\omegaT}', 'texmode', 'on')
  "Delay_1 " : Subsystem
      mask Display: disp('\fontname{Times New Roman}\ite^{-j\omegaT}', 'texmode', 'on')
  E_1 : Subsystem
      mask Display: disp('\fontname{Times New Roman}\fontsize{30}\itE', 'texmode', 'on')
  E_2 : Subsystem
      mask Display: disp('\fontname{Times New Roman}\fontsize{30}\itE', 'texmode', 'on')
  F_1 : Subsystem
      mask Display: disp('\fontname{Times New Roman}\fontsize{30}\itF', 'texmode', 'on')
  F_2 : Subsystem
      mask Display: disp('\fontname{Times New Roman}\fontsize{30}\itF', 'texmode', 'on')
  G_1 : Subsystem
      mask Display: disp('\fontname{Times New Roman}\fontsize{30}\itG', 'texmode', 'on')
  G_2 : Subsystem
      mask Display: disp('\fontname{Times New Roman}\fontsize{30}\itG', 'texmode', 'on')
  Gain2 : Gain  Gain=1/Z_c
  Gain3 : Gain  Gain=1/Z_c
  Sum : Sum  Inputs=|++
  Sum1 : Sum  Inputs=|++
  Sum2 : Sum  Inputs=++|
  Sum3 : Sum  Inputs=++|
  Sum5 : Sum  Inputs=-+|
  Sum6 : Sum  Inputs=|+-
  Q_1 : Outport
  Q_2 : Outport  Port=2
  wires:
  Sum2/1 -> Sum6/2
  Gain2/1 -> E_1/1(Q_1), F_1/1(Q_1), Q_1/1
  Sum6/1 -> Gain2/1
  P_1/1 -> Sum/1, Sum6/1
  F_1/1(F) -> Sum/2
  Sum5/1 -> Gain3/1
  Gain3/1 -> Q_2/1, E_2/1(Q_2), F_2/2(Q_2)
  "  Delay_2 "/1(delay) -> Sum2/2
  "Delay_1 "/1(delay) -> Sum1/1
  P_2/1 -> Sum3/2, Sum5/2
  Sum1/1 -> Sum5/1
  F_2/1(F) -> Sum3/1
  Sum3/1 -> G_2/1(F + P_2)
  G_2/1(G) -> "  Delay_2 "/1(G)
  E_1/1(E) -> Sum2/1, F_1/2(E)
  E_2/1(E) -> F_2/1(E), Sum1/2
  G_1/1(G) -> "Delay_1 "/1(G)
  Sum/1 -> G_1/1(F + P_1)

== system usask_tlm_lib/TLM Johnston P1P2/E2 ==
  In : Inport
  Transfer Fcn : TransferFcn  Numerator=[R]  Denominator=[K*T 1]
  Out : Outport
  wires:
  Transfer Fcn/1 -> Out/1
  In/1 -> Transfer Fcn/1

== system usask_tlm_lib/TLM Johnston P1P2/F2 ==
  In : Inport
  Gain : Gain  Gain=Zc
  Out : Outport
  wires:
  Gain/1 -> Out/1
  In/1 -> Gain/1

== system usask_tlm_lib/TLM Johnston P1P2/G1 ==
  In : Inport
  G2 : Subsystem  mask(Johnston G2){modelNumber=modelNumber}
      mask prompts: modelNumber "Model"
      mask help: This implements Johnston's G2 models. Model may be 1, 2 or 3 (see paper). Model 1 may be unstable for large beta.
      mask init:
      | k=4;%this must match order of diagram
      | m=nan(k,1);
      | m(1)=2.2457;
      | if k>1
      | m(2)=6.8400;
      | end
      | for i=3:k
      |     m(i)=3*m(i-1);
      | end
      | 
      | 
      | n=nan(k,1);
      | n(1)=42.849;
      | for i=2:k
      |     n(i)=9*n(i-1);
      | end
      | 
      | 
      | if modelNumber==1
      |         bypass1=false;
      |         bypass2=true;
      |         numGain=2;%numerator gain
      | elseif modelNumber==2
      |     bypass1=true;
      |         bypass2=false;
      |         numGain=2;%numerator gain
      | elseif modelNumber==3
      |         bypass1=false;
      |         bypass2=false;
      |         numGain=1;%numerator gain
      | else
      |     warning('Model number must be 1, 2, or 3')
      | end
  Transfer Fcn : TransferFcn  Numerator=[K*beta*r^2/nu*exp(-4*beta) 1]  Denominator=[K*beta*r^2/nu 1]
  Out : Outport
  wires:
  In/1 -> Transfer Fcn/1
  Transfer Fcn/1 -> G2/1(In)
  G2/1(Out) -> Out/1

== system usask_tlm_lib/TLM Johnston P1P2/G2 ==
  In : Inport
  G2 : Subsystem  mask(Johnston G2){modelNumber=modelNumber}
      mask prompts: modelNumber "Model"
      mask help: This implements Johnston's G2 models. Model may be 1, 2 or 3 (see paper). Model 1 may be unstable for large beta.
      mask init: same as usask_tlm_lib/TLM Johnston P1P2/G1/G2
  Transfer Fcn : TransferFcn  Numerator=[K*beta*r^2/nu*exp(-4*beta) 1]  Denominator=[K*beta*r^2/nu 1]
  Out : Outport
  wires:
  In/1 -> Transfer Fcn/1
  Transfer Fcn/1 -> G2/1(In)
  G2/1(Out) -> Out/1

== system usask_tlm_lib/TLM Johnston P1Q2/Ea ==
  In : Inport
  Transfer Fcn : TransferFcn  Numerator=[R]  Denominator=[K*T 1]
  Out : Outport
  wires:
  In/1 -> Transfer Fcn/1
  Transfer Fcn/1 -> Out/1

== system usask_tlm_lib/TLM Johnston P1Q2/Eb ==
  In : Inport
  Transfer Fcn : TransferFcn  Numerator=[R]  Denominator=[K*T 1]
  Out : Outport
  wires:
  In/1 -> Transfer Fcn/1
  Transfer Fcn/1 -> Out/1

== system usask_tlm_lib/TLM Johnston P1Q2/Fa ==
  In : Inport
  Gain : Gain  Gain=Zc
  Out : Outport
  wires:
  In/1 -> Gain/1
  Gain/1 -> Out/1

== system usask_tlm_lib/TLM Johnston P1Q2/Fb ==
  In : Inport
  Gain : Gain  Gain=Zc
  Out : Outport
  wires:
  In/1 -> Gain/1
  Gain/1 -> Out/1

== system usask_tlm_lib/TLM Johnston P1Q2/Ga ==
  In : Inport
  G2 : Subsystem  mask(Johnston G2){modelNumber=modelNumber}
      mask prompts: modelNumber "Model"
      mask help: This implements Johnston's G2 models. Model may be 1, 2 or 3 (see paper). Model 1 may be unstable for large beta.
      mask init: same as usask_tlm_lib/TLM Johnston P1P2/G1/G2
  Transfer Fcn : TransferFcn  Numerator=[K*beta*r^2/nu*exp(-4*beta) 1]  Denominator=[K*beta*r^2/nu 1]
  Out : Outport
  wires:
  G2/1(Out) -> Out/1
  Transfer Fcn/1 -> G2/1(In)
  In/1 -> Transfer Fcn/1

== system usask_tlm_lib/TLM Johnston P1Q2/Gb ==
  In : Inport
  G2 : Subsystem  mask(Johnston G2){modelNumber=modelNumber}
      mask prompts: modelNumber "Model"
      mask help: This implements Johnston's G2 models. Model may be 1, 2 or 3 (see paper). Model 1 may be unstable for large beta.
      mask init: same as usask_tlm_lib/TLM Johnston P1P2/G1/G2
  Transfer Fcn : TransferFcn  Numerator=[K*beta*r^2/nu*exp(-4*beta) 1]  Denominator=[K*beta*r^2/nu 1]
  Out : Outport
  wires:
  G2/1(Out) -> Out/1
  Transfer Fcn/1 -> G2/1(In)
  In/1 -> Transfer Fcn/1

== system usask_tlm_lib/TLM Johnston Q1P2/Ea ==
  In : Inport
  Transfer Fcn : TransferFcn  Numerator=[R]  Denominator=[K*T 1]
  Out : Outport
  wires:
  In/1 -> Transfer Fcn/1
  Transfer Fcn/1 -> Out/1

== system usask_tlm_lib/TLM Johnston Q1P2/Eb ==
  In : Inport
  Transfer Fcn : TransferFcn  Numerator=[R]  Denominator=[K*T 1]
  Out : Outport
  wires:
  In/1 -> Transfer Fcn/1
  Transfer Fcn/1 -> Out/1

== system usask_tlm_lib/TLM Johnston Q1P2/Fa ==
  In : Inport
  Gain : Gain  Gain=Zc
  Out : Outport
  wires:
  In/1 -> Gain/1
  Gain/1 -> Out/1

== system usask_tlm_lib/TLM Johnston Q1P2/Fb ==
  In : Inport
  Gain : Gain  Gain=Zc
  Out : Outport
  wires:
  In/1 -> Gain/1
  Gain/1 -> Out/1

== system usask_tlm_lib/TLM Johnston Q1P2/Ga ==
  In : Inport
  G2 : Subsystem  mask(Johnston G2){modelNumber=modelNumber}
      mask prompts: modelNumber "Model"
      mask help: This implements Johnston's G2 models. Model may be 1, 2 or 3 (see paper). Model 1 may be unstable for large beta.
      mask init: same as usask_tlm_lib/TLM Johnston P1P2/G1/G2
  Transfer Fcn : TransferFcn  Numerator=[K*beta*r^2/nu*exp(-4*beta) 1]  Denominator=[K*beta*r^2/nu 1]
  Out : Outport
  wires:
  G2/1(Out) -> Out/1
  Transfer Fcn/1 -> G2/1(In)
  In/1 -> Transfer Fcn/1

== system usask_tlm_lib/TLM Johnston Q1P2/Gb ==
  In : Inport
  G2 : Subsystem  mask(Johnston G2){modelNumber=modelNumber}
      mask prompts: modelNumber "Model"
      mask help: This implements Johnston's G2 models. Model may be 1, 2 or 3 (see paper). Model 1 may be unstable for large beta.
      mask init: same as usask_tlm_lib/TLM Johnston P1P2/G1/G2
  Transfer Fcn : TransferFcn  Numerator=[K*beta*r^2/nu*exp(-4*beta) 1]  Denominator=[K*beta*r^2/nu 1]
  Out : Outport
  wires:
  G2/1(Out) -> Out/1
  Transfer Fcn/1 -> G2/1(In)
  In/1 -> Transfer Fcn/1

== system usask_tlm_lib/TLM Johnston Q1Q2/Ea ==
  In : Inport
  Transfer Fcn : TransferFcn  Numerator=[R]  Denominator=[K*T 1]
  Out : Outport
  wires:
  In/1 -> Transfer Fcn/1
  Transfer Fcn/1 -> Out/1

== system usask_tlm_lib/TLM Johnston Q1Q2/Eb ==
  In : Inport
  Transfer Fcn : TransferFcn  Numerator=[R]  Denominator=[K*T 1]
  Out : Outport
  wires:
  In/1 -> Transfer Fcn/1
  Transfer Fcn/1 -> Out/1

== system usask_tlm_lib/TLM Johnston Q1Q2/Fa ==
  In : Inport
  Gain : Gain  Gain=Zc
  Out : Outport
  wires:
  In/1 -> Gain/1
  Gain/1 -> Out/1

== system usask_tlm_lib/TLM Johnston Q1Q2/Fb ==
  In : Inport
  Gain : Gain  Gain=Zc
  Out : Outport
  wires:
  In/1 -> Gain/1
  Gain/1 -> Out/1

== system usask_tlm_lib/TLM Johnston Q1Q2/Ga ==
  In : Inport
  G2 : Subsystem  mask(Johnston G2){modelNumber=modelNumber}
      mask prompts: modelNumber "Model"
      mask help: This implements Johnston's G2 models. Model may be 1, 2 or 3 (see paper). Model 1 may be unstable for large beta.
      mask init: same as usask_tlm_lib/TLM Johnston P1P2/G1/G2
  Transfer Fcn : TransferFcn  Numerator=[K*beta*r^2/nu*exp(-4*beta) 1]  Denominator=[K*beta*r^2/nu 1]
  Out : Outport
  wires:
  G2/1(Out) -> Out/1
  Transfer Fcn/1 -> G2/1(In)
  In/1 -> Transfer Fcn/1

== system usask_tlm_lib/TLM Johnston Q1Q2/Gb ==
  In : Inport
  G2 : Subsystem  mask(Johnston G2){modelNumber=modelNumber}
      mask prompts: modelNumber "Model"
      mask help: This implements Johnston's G2 models. Model may be 1, 2 or 3 (see paper). Model 1 may be unstable for large beta.
      mask init: same as usask_tlm_lib/TLM Johnston P1P2/G1/G2
  Transfer Fcn : TransferFcn  Numerator=[K*beta*r^2/nu*exp(-4*beta) 1]  Denominator=[K*beta*r^2/nu 1]
  Out : Outport
  wires:
  G2/1(Out) -> Out/1
  Transfer Fcn/1 -> G2/1(In)
  In/1 -> Transfer Fcn/1

== system usask_tlm_lib/TLM Krus P1P2/E1 ==
  In : Inport
  Transfer Fcn : TransferFcn  Numerator=[R]  Denominator=[K*T 1]
  Out : Outport
  wires:
  Transfer Fcn/1 -> Out/1
  In/1 -> Transfer Fcn/1

== system usask_tlm_lib/TLM Krus P1P2/E2 ==
  In : Inport
  Transfer Fcn : TransferFcn  Numerator=[R]  Denominator=[K*T 1]
  Out : Outport
  wires:
  Transfer Fcn/1 -> Out/1
  In/1 -> Transfer Fcn/1

== system usask_tlm_lib/TLM Krus P1P2/F1 ==
  In : Inport
  Gain : Gain  Gain=Zc
  Out : Outport
  wires:
  Gain/1 -> Out/1
  In/1 -> Gain/1

== system usask_tlm_lib/TLM Krus P1P2/F2 ==
  In : Inport
  Gain : Gain  Gain=Zc
  Out : Outport
  wires:
  Gain/1 -> Out/1
  In/1 -> Gain/1

== system usask_tlm_lib/TLM Krus P1P2/G1 ==
  In : Inport
  Transfer Fcn : TransferFcn  Numerator=[K*T*exp(-R*A/(2*rho*c)) 1]  Denominator=[K*T 1]
  Out : Outport
  wires:
  Transfer Fcn/1 -> Out/1
  In/1 -> Transfer Fcn/1

== system usask_tlm_lib/TLM Krus P1P2/G2 ==
  In : Inport
  Transfer Fcn : TransferFcn  Numerator=[K*T*exp(-R*A/(2*rho*c)) 1]  Denominator=[K*T 1]
  Out : Outport
  wires:
  Transfer Fcn/1 -> Out/1
  In/1 -> Transfer Fcn/1

== system usask_tlm_lib/TLM Krus P1Q2/E1 ==
  In : Inport
  Transfer Fcn : TransferFcn  Numerator=[R]  Denominator=[K*T 1]
  Out : Outport
  wires:
  In/1 -> Transfer Fcn/1
  Transfer Fcn/1 -> Out/1

== system usask_tlm_lib/TLM Krus P1Q2/E2 ==
  In : Inport
  Transfer Fcn : TransferFcn  Numerator=[R]  Denominator=[K*T 1]
  Out : Outport
  wires:
  In/1 -> Transfer Fcn/1
  Transfer Fcn/1 -> Out/1

== system usask_tlm_lib/TLM Krus P1Q2/F1 ==
  In : Inport
  Gain : Gain  Gain=Zc
  Out : Outport
  wires:
  In/1 -> Gain/1
  Gain/1 -> Out/1

== system usask_tlm_lib/TLM Krus P1Q2/F2 ==
  In : Inport
  Gain : Gain  Gain=Zc
  Out : Outport
  wires:
  In/1 -> Gain/1
  Gain/1 -> Out/1

== system usask_tlm_lib/TLM Krus P1Q2/G1 ==
  In : Inport
  Transfer Fcn : TransferFcn  Numerator=[K*T*exp(-R*A/(2*rho*c)) 1]  Denominator=[K*T 1]
  Out : Outport
  wires:
  In/1 -> Transfer Fcn/1
  Transfer Fcn/1 -> Out/1

== system usask_tlm_lib/TLM Krus P1Q2/G2 ==
  In : Inport
  Transfer Fcn : TransferFcn  Numerator=[K*T*exp(-R*A/(2*rho*c)) 1]  Denominator=[K*T 1]
  Out : Outport
  wires:
  In/1 -> Transfer Fcn/1
  Transfer Fcn/1 -> Out/1

== system usask_tlm_lib/TLM Krus Q1P2/E1 ==
  In : Inport
  Transfer Fcn : TransferFcn  Numerator=[R]  Denominator=[K*T 1]
  Out : Outport
  wires:
  Transfer Fcn/1 -> Out/1
  In/1 -> Transfer Fcn/1

== system usask_tlm_lib/TLM Krus Q1P2/E2 ==
  In : Inport
  Transfer Fcn : TransferFcn  Numerator=[R]  Denominator=[K*T 1]
  Out : Outport
  wires:
  Transfer Fcn/1 -> Out/1
  In/1 -> Transfer Fcn/1

== system usask_tlm_lib/TLM Krus Q1P2/F1 ==
  In : Inport
  Gain : Gain  Gain=Zc
  Out : Outport
  wires:
  Gain/1 -> Out/1
  In/1 -> Gain/1

== system usask_tlm_lib/TLM Krus Q1P2/F2 ==
  In : Inport
  Gain : Gain  Gain=Zc
  Out : Outport
  wires:
  Gain/1 -> Out/1
  In/1 -> Gain/1

== system usask_tlm_lib/TLM Krus Q1P2/G1 ==
  In : Inport
  Transfer Fcn : TransferFcn  Numerator=[K*T*exp(-R*A/(2*rho*c)) 1]  Denominator=[K*T 1]
  Out : Outport
  wires:
  Transfer Fcn/1 -> Out/1
  In/1 -> Transfer Fcn/1

== system usask_tlm_lib/TLM Krus Q1P2/G2 ==
  In : Inport
  Transfer Fcn : TransferFcn  Numerator=[K*T*exp(-R*A/(2*rho*c)) 1]  Denominator=[K*T 1]
  Out : Outport
  wires:
  Transfer Fcn/1 -> Out/1
  In/1 -> Transfer Fcn/1

== system usask_tlm_lib/TLM Krus Q1Q2/E1 ==
  In : Inport
  Transfer Fcn : TransferFcn  Numerator=[R]  Denominator=[K*T 1]
  Out : Outport
  wires:
  Transfer Fcn/1 -> Out/1
  In/1 -> Transfer Fcn/1

== system usask_tlm_lib/TLM Krus Q1Q2/E2 ==
  In : Inport
  Transfer Fcn : TransferFcn  Numerator=[R]  Denominator=[K*T 1]
  Out : Outport
  wires:
  Transfer Fcn/1 -> Out/1
  In/1 -> Transfer Fcn/1

== system usask_tlm_lib/TLM Krus Q1Q2/F1 ==
  In : Inport
  Gain : Gain  Gain=Zc
  Out : Outport
  wires:
  Gain/1 -> Out/1
  In/1 -> Gain/1

== system usask_tlm_lib/TLM Krus Q1Q2/F2 ==
  In : Inport
  Gain : Gain  Gain=Zc
  Out : Outport
  wires:
  Gain/1 -> Out/1
  In/1 -> Gain/1

== system usask_tlm_lib/TLM Krus Q1Q2/G1 ==
  In : Inport
  Transfer Fcn : TransferFcn  Numerator=[K*T*exp(-R*A/(2*rho*c)) 1]  Denominator=[K*T 1]
  Out : Outport
  wires:
  Transfer Fcn/1 -> Out/1
  In/1 -> Transfer Fcn/1

== system usask_tlm_lib/TLM Krus Q1Q2/G2 ==
  In : Inport
  Transfer Fcn : TransferFcn  Numerator=[K*T*exp(-R*A/(2*rho*c)) 1]  Denominator=[K*T 1]
  Out : Outport
  wires:
  Transfer Fcn/1 -> Out/1
  In/1 -> Transfer Fcn/1

== system usask_tlm_lib/Tapered TLM P1P2/  Delay_2  ==
  G : Inport
  Transport Delay : TransportDelay  DelayTime=T_prime
  delay : Outport
  wires:
  Transport Delay/1 -> delay/1
  G/1 -> Transport Delay/1

== system usask_tlm_lib/Tapered TLM P1P2/Delay_1  ==
  G : Inport
  Transport Delay : TransportDelay  DelayTime=T_prime
  delay : Outport
  wires:
  Transport Delay/1 -> delay/1
  G/1 -> Transport Delay/1

== system usask_tlm_lib/Tapered TLM P1P2/E_1 ==
  note: Equation (14) from ven der Buhs et al. 2017
  Q_1 : Inport
  Gain : Gain  Gain=Z_c
  Sum : Sum  Inputs=++++++
  k = 1 : TransferFcn  Numerator=[m_E(1)]  Denominator=[T n(1)]
  k = 2 : TransferFcn  Numerator=[m_E(2)]  Denominator=[T n(2)]
  k = 3 : TransferFcn  Numerator=[m_E(3)]  Denominator=[T n(3)]
  k = 4 : TransferFcn  Numerator=[m_E(4)]  Denominator=[T n(4)]
  k = 5 : TransferFcn  Numerator=[m_E(5)]  Denominator=[T n(5)]
  k = 6 : TransferFcn  Numerator=[m_E(6)]  Denominator=[T n(6)]
  E : Outport
  wires:
  Q_1/1 -> k = 4/1, k = 5/1, k = 6/1, k = 3/1, k = 1/1, k = 2/1
  k = 6/1 -> Sum/6
  k = 5/1 -> Sum/5
  k = 4/1 -> Sum/4
  k = 3/1 -> Sum/3
  k = 2/1 -> Sum/2
  k = 1/1 -> Sum/1
  Sum/1 -> Gain/1
  Gain/1 -> E/1

== system usask_tlm_lib/Tapered TLM P1P2/E_2 ==
  note: Equation (14) from ven der Buhs et al. 2017
  Q_2 : Inport
  Gain : Gain  Gain=Z_c
  Sum : Sum  Inputs=++++++
  k = 1 : TransferFcn  Numerator=[m_E(1)]  Denominator=[T n(1)]
  k = 2 : TransferFcn  Numerator=[m_E(2)]  Denominator=[T n(2)]
  k = 3 : TransferFcn  Numerator=[m_E(3)]  Denominator=[T n(3)]
  k = 4 : TransferFcn  Numerator=[m_E(4)]  Denominator=[T n(4)]
  k = 5 : TransferFcn  Numerator=[m_E(5)]  Denominator=[T n(5)]
  k = 6 : TransferFcn  Numerator=[m_E(6)]  Denominator=[T n(6)]
  E : Outport
  wires:
  Q_2/1 -> k = 4/1, k = 5/1, k = 6/1, k = 3/1, k = 1/1, k = 2/1
  k = 6/1 -> Sum/6
  k = 5/1 -> Sum/5
  k = 4/1 -> Sum/4
  k = 3/1 -> Sum/3
  k = 2/1 -> Sum/2
  k = 1/1 -> Sum/1
  Sum/1 -> Gain/1
  Gain/1 -> E/1

== system usask_tlm_lib/Tapered TLM P1P2/F_1 ==
  note: Equation (15) from ven der Buhs et al. 2017
  Q_1 : Inport
  E : Inport  Port=2
  Gain : Gain  Gain=b
  Gain1 : Gain  Gain=Z_c
  Sum : Sum
  Out1 : Outport
  wires:
  E/1 -> Gain/1
  Q_1/1 -> Gain1/1
  Sum/1 -> Out1/1
  Gain1/1 -> Sum/1
  Gain/1 -> Sum/2

== system usask_tlm_lib/Tapered TLM P1P2/F_2 ==
  note: Equation (15) from ven der Buhs et al. 2017
  E : Inport
  Q_2 : Inport  Port=2
  Gain : Gain  Gain=b
  Gain1 : Gain  Gain=Z_c
  Sum : Sum
  F : Outport
  wires:
  Gain/1 -> Sum/2
  Gain1/1 -> Sum/1
  Sum/1 -> F/1
  Q_2/1 -> Gain1/1
  E/1 -> Gain/1
